simulink model "PIC32MK_MCPWM_MCLV2_PIM_SingleShunt_R2015b_InternalOpAmp"  (R2015b)
settings: Solver=FixedStepDiscrete  StartTime=0.0  StopTime=1  FixedStep=5e-5  RelTol=1e-3
undefined symbols (not defined in the file): A0, A11, A4, AN24, AN25, AN6, AN9, B6, B7, B9, C0, C8, DiscIntNeverNeededParam, G15, MaxPer, ms, Pin, PWM1max, Resol, us, XData
libraries: MCHP_Blockset x14, simulink x9
(part 2 of 3)

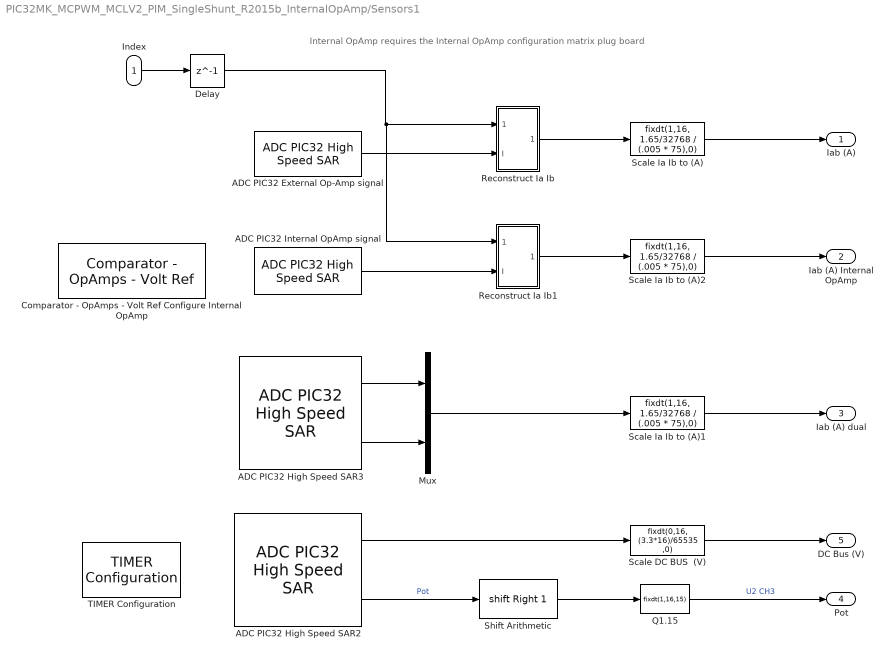
== system PIC32MK_MCPWM_MCLV2_PIM_SingleShunt_R2015b_InternalOpAmp/Sensors1 ==
  note: Internal OpAmp requires the Internal OpAmp configuration matrix plug board
  Index : Inport
  "ADC PIC32 External Op-Amp signal " : MCHP_Blockset/Analog IO/ADC PIC32 High Speed SAR  Priority=-5000  ADC_VrefH=AVdd (default)  ADC_VrefL=AVss (default)  ADC_FRACT=Fractional (left aligned)  DMA_Size=2 trig / 2 elements output (use DMA ping-pong buffer)  ADC_Synchronisation=Triggered by custom source  ADC_Trig=Dynamic Options  ADC_Trig_TXT=PWM1 trigger  ADC_TrigTimeStep=on  ADC_TrigInfo=0  SampleTime=.00005  S_INPUT=[]  S_INPUT_Size=[]  S_OUTPUT=[4]  S_OUTPUT_Size=[2]  S_ListCustomDatatype=S.S_ListCustomDatatype={};  MCHP_USER_INTERRUPTS={AD1D5}{ADC5Data}{ADC Data 5 Ready}{VectorName(ADC_DATA5_VECTOR) Priority(-1) Config_BitSet(ADCGIRQEN1bits.AGIEN5) RegisterReadClear(ADCDATA5)};  MCHP_PORT={Analog Input 25}{AN25}15:2:B7;  MCHP_MASTERLINK=PIC32MK_MCPWM_MCLV2_PIM_SingleShunt_R2015a_InternalOpAmp/Microchip Master  MCHP_CRC=2653067  ADC_Info=Total Time = 450(ns)  ADC0_pin=Dynamic Options  ADC0_pin_TXT=Not used  ADC0_R=< 200 Ohm  ADC0_res=12 bits  ADC0_signed=signed 16 bits  ADC0_FILTER=No Oversampling  ADC0_FILTER_nSamples=8 samples  ADC0_STRGEN=End sampling and start conversion  ADC0_SSAMPEN=on  ADC0_Info=tSmp_min=33.333(ns) x -1 = -33.333(ns) ; tConv=166.67(ns) x 0 = 0(s) ; TOTAL=0(s)  ADC1_pin=Dynamic Options  ADC1_pin_TXT=Not used  ADC1_R=< 200 Ohm  ADC1_res=12 bits  ADC1_signed=signed 16 bits  ADC1_FILTER=No Oversampling  ADC1_FILTER_nSamples=256 samples  ADC1_STRGEN=End sampling and start conversion  ADC1_SSAMPEN=on  ADC1_Info=tSmp_min=33.333(ns) x -1 = -33.333(ns) ; tConv=166.67(ns) x 0 = 0(s) ; TOTAL=0(s)  ADC2_pin=Dynamic Options  ADC2_pin_TXT=Not used  ADC2_R=< 200 Ohm  ADC2_res=12 bits  ADC2_signed=signed 16 bits  ADC2_FILTER=No Oversampling  ADC2_FILTER_nSamples=256 samples  ADC2_STRGEN=End sampling and start conversion  ADC2_SSAMPEN=off  ADC2_Info=tSmp_min=33.333(ns) x -1 = -33.333(ns) ; tConv=166.67(ns) x 0 = 0(s) ; TOTAL=0(s)  ADC3_pin=Dynamic Options  ADC3_pin_TXT=Not used  ADC3_R=< 200 Ohm  ADC3_res=12 bits  ADC3_signed=unsigned 16 bits  ADC3_FILTER=No Oversampling  ADC3_FILTER_nSamples=256 samples  ADC3_STRGEN=End sampling and start conversion  ADC3_SSAMPEN=on  ADC3_Info=tSmp_min=33.333(ns) x -1 = -33.333(ns) ; tConv=166.67(ns) x 0 = 0(s) ; TOTAL=0(s)  ADC4_pin=Dynamic Options  ADC4_pin_TXT=Not used  ADC4_R=< 200 Ohm  ADC4_res=12 bits  ADC4_signed=unsigned 16 bits  ADC4_FILTER=Burst convert of n samples are Averaged  ADC4_FILTER_nSamples=256 samples  ADC4_STRGEN=End sampling and start conversion  ADC4_SSAMPEN=off  ADC4_Info=tSmp_min=33.333(ns) x -1 = -33.333(ns) ; tConv=166.67(ns) x 0 = 0(s) ; TOTAL=0(s)  ADC5_pin=Dynamic Options  ADC5_pin_TXT=AN25 / B7 / Pin[72]  ADC5_R=< 200 Ohm  ADC5_res=12 bits  ADC5_signed=signed 16 bits  ADC5_FILTER=No Oversampling  ADC5_FILTER_nSamples=256 samples  ADC5_STRGEN=End sampling and start conversion  ADC5_SSAMPEN=off  ADC5_Info=tSmp_min=100(ns) x 0 = 0(s) ; tConv=433.33(ns) x 1 = 433.33(ns) ; TOTAL=450(ns)  ADC6_pin=Dynamic Options  ADC6_pin_TXT=Not used  ADC6_R=< 200 Ohm  ADC6_res=12 bits  ADC6_signed=unsigned 16 bits  ADC6_FILTER=Burst convert of n samples are Summed  ADC6_FILTER_nSamples=256 samples  ADC6_STRGEN=End sampling and start conversion  ADC6_SSAMPEN=on  ADC6_Info=tSmp_min=33.333(ns) x -1 = -33.333(ns) ; tConv=166.67(ns) x 0 = 0(s) ; TOTAL=0(s)  ADC7_R=< 200 Ohm  ADC7_res=12 bits  ADC7_AN0=Not used  ADC7_AN1=Not used  ADC7_AN2=Not used  ADC7_AN3=Not used  ADC7_AN4=Not used  ADC7_AN5=Not used  ADC7_AN6=Not used  ADC7_AN7=Not used  ADC7_AN8=Not used  ADC7_AN9=Not used  ADC7_AN10=Not used  ADC7_AN11=Not used  ADC7_AN12=Not used  ADC7_AN13=Not used  ADC7_AN14=Not used  ADC7_AN15=Not used  ADC7_AN16=Not used  ADC7_AN17=Not used  ADC7_AN18=Not used  ADC7_AN19=Not used  ADC7_AN20=Not used  ADC7_AN21=Not used  ADC7_AN22=Not used  ADC7_AN23=Not used  ADC7_AN24=Not used  ADC7_AN25=Not used  ADC7_AN26=Not used  ADC7_AN27=Not used  ADC7_AN28=Not used  ADC7_AN29=Not used  ADC7_AN30=Not used  ADC7_AN31=Not used  ADC7_AN32=Not used  ADC7_AN33=Not used  ADC7_AN34=Not used  ADC7_AN35=Not used  ADC7_AN36=Not used  ADC7_AN37=Not used  ADC7_AN38=Not used  ADC7_AN39=Not used  ADC7_AN40=Not used  ADC7_AN41=Not used  ADC7_AN42=Not used  ADC7_AN43=Not used  ADC7_AN44=Not used  ADC7_AN45=Not used  ADC7_AN46=Not used  ADC7_AN47=Not used  ADC7_AN48=Not used  ADC7_AN49=Not used  ADC7_AN50=Not used  ADC7_AN51=Not used  ADC7_AN52=Not used  ADC7_AN53=Not used  ADC7_AN54=Not used  ADC7_AN55=Not used  ADC7_AN56=Not used  ADC7_AN57=Not used  ADC7_AN58=Not used  ADC7_AN59=Not used  ADC7_AN60=Not used  ADC7_AN61=Not used  ADC7_AN62=Not used  ADC7_AN63=Not used  CTMU_Temp=Not used  Vbat=Not used  IVref=Not used  IVTemp=Not used
  ADC PIC32 High Speed SAR2 : MCHP_Blockset/Analog IO/ADC PIC32 High Speed SAR  Priority=-5000  ADC_VrefH=AVdd (default)  ADC_VrefL=AVss (default)  ADC_FRACT=Fractional (left aligned)  DMA_Size=Single trigger - (no DMA)  ADC_Synchronisation=Triggered by custom source  ADC_Trig=Dynamic Options  ADC_Trig_TXT=TMR5 Match  ADC_TrigTimeStep=off  ADC_TrigInfo=0  SampleTime=.001  S_INPUT=[]  S_INPUT_Size=[]  S_OUTPUT="[5  5]"  S_OUTPUT_Size="[1  1]"  S_ListCustomDatatype=S.S_ListCustomDatatype={};  MCHP_USER_INTERRUPTS={AD1D9}{ADC9Data}{ADC Data 9 Ready}{VectorName(ADC_DATA9_VECTOR) Priority(-1) Config_BitSet(ADCGIRQEN1bits.AGIEN9) RegisterReadClear(ADCDATA9)};{AD1D14}{ADC14Data}{ADC Data 14 Ready}{VectorName(ADC_DATA14_VECTOR) Priority(-1) Config_BitSet(ADCGIRQEN1bits.AGIEN14) RegisterReadClear(ADCDATA14)};  MCHP_PORT={Analog Input 10}{AN10}15:2:A12;{Analog Input 15}{AN15}15:2:E15;  MCHP_MASTERLINK=PIC32MK_MCPWM_MCLV2_PIM_SingleShunt_R2015a_InternalOpAmp/Microchip Master  MCHP_CRC=2878404  ADC_Info=Total Time = 149.917(us)  ADC0_pin=Dynamic Options  ADC0_pin_TXT=Not used  ADC0_R=< 200 Ohm  ADC0_res=12 bits  ADC0_signed=signed 16 bits  ADC0_FILTER=No Oversampling  ADC0_FILTER_nSamples=256 samples  ADC0_STRGEN=End sampling and start conversion  ADC0_SSAMPEN=on  ADC0_Info=tSmp_min=33.333(ns) x -1 = -33.333(ns) ; tConv=166.67(ns) x 0 = 0(s) ; TOTAL=0(s)  ADC1_pin=Dynamic Options  ADC1_pin_TXT=Not used  ADC1_R=< 200 Ohm  ADC1_res=12 bits  ADC1_signed=signed 16 bits  ADC1_FILTER=No Oversampling  ADC1_FILTER_nSamples=256 samples  ADC1_STRGEN=End sampling and start conversion  ADC1_SSAMPEN=on  ADC1_Info=tSmp_min=33.333(ns) x -1 = -33.333(ns) ; tConv=166.67(ns) x 0 = 0(s) ; TOTAL=0(s)  ADC2_pin=Dynamic Options  ADC2_pin_TXT=Not used  ADC2_R=< 200 Ohm  ADC2_res=12 bits  ADC2_signed=signed 16 bits  ADC2_FILTER=Burst convert of n samples are Summed  ADC2_FILTER_nSamples=256 samples  ADC2_STRGEN=End sampling and start conversion  ADC2_SSAMPEN=off  ADC2_Info=tSmp_min=33.333(ns) x -1 = -33.333(ns) ; tConv=166.67(ns) x 0 = 0(s) ; TOTAL=0(s)  ADC3_pin=Dynamic Options  ADC3_pin_TXT=Not used  ADC3_R=< 200 Ohm  ADC3_res=12 bits  ADC3_signed=unsigned 16 bits  ADC3_FILTER=No Oversampling  ADC3_FILTER_nSamples=256 samples  ADC3_STRGEN=End sampling and start conversion  ADC3_SSAMPEN=on  ADC3_Info=tSmp_min=33.333(ns) x -1 = -33.333(ns) ; tConv=166.67(ns) x 0 = 0(s) ; TOTAL=0(s)  ADC4_pin=Dynamic Options  ADC4_pin_TXT=Not used  ADC4_R=< 200 Ohm  ADC4_res=12 bits  ADC4_signed=unsigned 16 bits  ADC4_FILTER=Burst convert of n samples are Averaged  ADC4_FILTER_nSamples=256 samples  ADC4_STRGEN=End sampling and start conversion  ADC4_SSAMPEN=off  ADC4_Info=tSmp_min=33.333(ns) x -1 = -33.333(ns) ; tConv=166.67(ns) x 0 = 0(s) ; TOTAL=0(s)  ADC5_pin=Dynamic Options  ADC5_pin_TXT=Not used  ADC5_R=< 200 Ohm  ADC5_res=12 bits  ADC5_signed=unsigned 16 bits  ADC5_FILTER=No Oversampling  ADC5_FILTER_nSamples=256 samples  ADC5_STRGEN=End sampling and start conversion  ADC5_SSAMPEN=off  ADC5_Info=tSmp_min=33.333(ns) x -1 = -33.333(ns) ; tConv=166.67(ns) x 0 = 0(s) ; TOTAL=0(s)  ADC6_pin=Dynamic Options  ADC6_pin_TXT=Not used  ADC6_R=< 200 Ohm  ADC6_res=12 bits  ADC6_signed=unsigned 16 bits  ADC6_FILTER=Burst convert of n samples are Summed  ADC6_FILTER_nSamples=256 samples  ADC6_STRGEN=End sampling and start conversion  ADC6_SSAMPEN=on  ADC6_Info=tSmp_min=33.333(ns) x -1 = -33.333(ns) ; tConv=166.67(ns) x 0 = 0(s) ; TOTAL=0(s)  ADC7_R=< 200 Ohm  ADC7_res=12 bits  ADC7_AN0=Not used  ADC7_AN1=Not used  ADC7_AN2=Not used  ADC7_AN3=Not used  ADC7_AN4=Not used  ADC7_AN5=Not used  ADC7_AN6=Not used  ADC7_AN7=Not used  ADC7_AN8=Not used  ADC7_AN9=Not used  ADC7_AN10=unsigned int16  ADC7_AN11=Not used  ADC7_AN12=Not used  ADC7_AN13=Not used  ADC7_AN14=Not used  ADC7_AN15=256 samples averaged - unsigned int16  ADC7_AN16=Not used  ADC7_AN17=Not used  ADC7_AN18=Not used  ADC7_AN19=Not used  ADC7_AN20=Not used  ADC7_AN21=Not used  ADC7_AN22=Not used  ADC7_AN23=Not used  ADC7_AN24=Not used  ADC7_AN25=Not used  ADC7_AN26=Not used  ADC7_AN27=Not used  ADC7_AN28=Not used  ADC7_AN29=Not used  ADC7_AN30=Not used  ADC7_AN31=Not used  ADC7_AN32=Not used  ADC7_AN33=Not used  ADC7_AN34=Not used  ADC7_AN35=Not used  ADC7_AN36=Not used  ADC7_AN37=Not used  ADC7_AN38=Not used  ADC7_AN39=Not used  ADC7_AN40=Not used  ADC7_AN41=Not used  ADC7_AN42=Not used  ADC7_AN43=Not used  ADC7_AN44=Not used  ADC7_AN45=Not used  ADC7_AN46=Not used  ADC7_AN47=Not used  ADC7_AN48=Not used  ADC7_AN49=Not used  ADC7_AN50=Not used  ADC7_AN51=Not used  ADC7_AN52=Not used  ADC7_AN53=Not used  ADC7_AN54=Not used  ADC7_AN55=Not used  ADC7_AN56=Not used  ADC7_AN57=Not used  ADC7_AN58=Not used  ADC7_AN59=Not used  ADC7_AN60=Not used  ADC7_AN61=Not used  ADC7_AN62=Not used  ADC7_AN63=Not used  CTMU_Temp=Not used  Vbat=Not used  IVref=Not used  IVTemp=Not used
  ADC PIC32 High Speed SAR3 : MCHP_Blockset/Analog IO/ADC PIC32 High Speed SAR  Priority=-5000  ADC_VrefH=AVdd (default)  ADC_VrefL=AVss (default)  ADC_FRACT=Fractional (left aligned)  DMA_Size=Single trigger - (no DMA)  ADC_Synchronisation=Triggered by custom source  ADC_Trig=Dynamic Options  ADC_Trig_TXT=PWM2 trigger  ADC_TrigTimeStep=off  ADC_TrigInfo=0  SampleTime=.00005  S_INPUT=[]  S_INPUT_Size=[]  S_OUTPUT="[4  4]"  S_OUTPUT_Size="[1  1]"  S_ListCustomDatatype=S.S_ListCustomDatatype={};  MCHP_USER_INTERRUPTS={AD1D0}{ADC0Data}{ADC Data 0 Ready}{VectorName(ADC_DATA0_VECTOR) Priority(-1) Config_BitSet(ADCGIRQEN1bits.AGIEN0) RegisterReadClear(ADCDATA0)};{AD1D4}{ADC4Data}{ADC Data 4 Ready}{VectorName(ADC_DATA4_VECTOR) Priority(-1) Config_BitSet(ADCGIRQEN1bits.AGIEN4) RegisterReadClear(ADCDATA4)};  MCHP_PORT={Analog Input 24}{AN24}15:2:A4;{Analog Input 9}{AN9}15:2:A11;  MCHP_MASTERLINK=PIC32MK_MCPWM_MCLV2_PIM_SingleShunt_R2015a_InternalOpAmp/Microchip Master  MCHP_CRC=2708506  ADC_Info=Total Time = 450(ns)  ADC0_pin=Dynamic Options  ADC0_pin_TXT=AN24 / A4 / Pin[51]  ADC0_R=< 200 Ohm  ADC0_res=12 bits  ADC0_signed=signed 16 bits  ADC0_FILTER=No Oversampling  ADC0_FILTER_nSamples=8 samples  ADC0_STRGEN=End sampling and start conversion  ADC0_SSAMPEN=on  ADC0_Info=tSmp_min=100(ns) x 0 = 0(s) ; tConv=433.33(ns) x 1 = 433.33(ns) ; TOTAL=450(ns)  ADC1_pin=Dynamic Options  ADC1_pin_TXT=Not used  ADC1_R=< 200 Ohm  ADC1_res=12 bits  ADC1_signed=signed 16 bits  ADC1_FILTER=No Oversampling  ADC1_FILTER_nSamples=256 samples  ADC1_STRGEN=End sampling and start conversion  ADC1_SSAMPEN=on  ADC1_Info=tSmp_min=33.333(ns) x -1 = -33.333(ns) ; tConv=166.67(ns) x 0 = 0(s) ; TOTAL=0(s)  ADC2_pin=Dynamic Options  ADC2_pin_TXT=Not used  ADC2_R=< 200 Ohm  ADC2_res=12 bits  ADC2_signed=signed 16 bits  ADC2_FILTER=No Oversampling  ADC2_FILTER_nSamples=256 samples  ADC2_STRGEN=End sampling and start conversion  ADC2_SSAMPEN=on  ADC2_Info=tSmp_min=33.333(ns) x -1 = -33.333(ns) ; tConv=166.67(ns) x 0 = 0(s) ; TOTAL=0(s)  ADC3_pin=Dynamic Options  ADC3_pin_TXT=Not used  ADC3_R=< 200 Ohm  ADC3_res=12 bits  ADC3_signed=unsigned 16 bits  ADC3_FILTER=No Oversampling  ADC3_FILTER_nSamples=256 samples  ADC3_STRGEN=End sampling and start conversion  ADC3_SSAMPEN=on  ADC3_Info=tSmp_min=33.333(ns) x -1 = -33.333(ns) ; tConv=166.67(ns) x 0 = 0(s) ; TOTAL=0(s)  ADC4_pin=Dynamic Options  ADC4_pin_TXT=AN9 / A11 / Pin[21]  ADC4_R=< 200 Ohm  ADC4_res=12 bits  ADC4_signed=signed 16 bits  ADC4_FILTER=No Oversampling  ADC4_FILTER_nSamples=256 samples  ADC4_STRGEN=End sampling and start conversion  ADC4_SSAMPEN=on  ADC4_Info=tSmp_min=100(ns) x 0 = 0(s) ; tConv=433.33(ns) x 1 = 433.33(ns) ; TOTAL=450(ns)  ADC5_pin=Dynamic Options  ADC5_pin_TXT=Not used  ADC5_R=< 200 Ohm  ADC5_res=12 bits  ADC5_signed=unsigned 16 bits  ADC5_FILTER=No Oversampling  ADC5_FILTER_nSamples=256 samples  ADC5_STRGEN=End sampling and start conversion  ADC5_SSAMPEN=off  ADC5_Info=tSmp_min=33.333(ns) x -1 = -33.333(ns) ; tConv=166.67(ns) x 0 = 0(s) ; TOTAL=0(s)  ADC6_pin=Dynamic Options  ADC6_pin_TXT=Not used  ADC6_R=< 200 Ohm  ADC6_res=12 bits  ADC6_signed=unsigned 16 bits  ADC6_FILTER=Burst convert of n samples are Summed  ADC6_FILTER_nSamples=256 samples  ADC6_STRGEN=End sampling and start conversion  ADC6_SSAMPEN=on  ADC6_Info=tSmp_min=33.333(ns) x -1 = -33.333(ns) ; tConv=166.67(ns) x 0 = 0(s) ; TOTAL=0(s)  ADC7_R=< 200 Ohm  ADC7_res=12 bits  ADC7_AN0=Not used  ADC7_AN1=Not used  ADC7_AN2=Not used  ADC7_AN3=Not used  ADC7_AN4=Not used  ADC7_AN5=Not used  ADC7_AN6=Not used  ADC7_AN7=Not used  ADC7_AN8=Not used  ADC7_AN9=Not used  ADC7_AN10=Not used  ADC7_AN11=Not used  ADC7_AN12=Not used  ADC7_AN13=Not used  ADC7_AN14=Not used  ADC7_AN15=Not used  ADC7_AN16=Not used  ADC7_AN17=Not used  ADC7_AN18=Not used  ADC7_AN19=Not used  ADC7_AN20=Not used  ADC7_AN21=Not used  ADC7_AN22=Not used  ADC7_AN23=Not used  ADC7_AN24=Not used  ADC7_AN25=Not used  ADC7_AN26=Not used  ADC7_AN27=Not used  ADC7_AN28=Not used  ADC7_AN29=Not used  ADC7_AN30=Not used  ADC7_AN31=Not used  ADC7_AN32=Not used  ADC7_AN33=Not used  ADC7_AN34=Not used  ADC7_AN35=Not used  ADC7_AN36=Not used  ADC7_AN37=Not used  ADC7_AN38=Not used  ADC7_AN39=Not used  ADC7_AN40=Not used  ADC7_AN41=Not used  ADC7_AN42=Not used  ADC7_AN43=Not used  ADC7_AN44=Not used  ADC7_AN45=Not used  ADC7_AN46=Not used  ADC7_AN47=Not used  ADC7_AN48=Not used  ADC7_AN49=Not used  ADC7_AN50=Not used  ADC7_AN51=Not used  ADC7_AN52=Not used  ADC7_AN53=Not used  ADC7_AN54=Not used  ADC7_AN55=Not used  ADC7_AN56=Not used  ADC7_AN57=Not used  ADC7_AN58=Not used  ADC7_AN59=Not used  ADC7_AN60=Not used  ADC7_AN61=Not used  ADC7_AN62=Not used  ADC7_AN63=Not used  CTMU_Temp=Not used  Vbat=Not used  IVref=Not used  IVTemp=Not used
  ADC PIC32 Internal OpAmp signal : MCHP_Blockset/Analog IO/ADC PIC32 High Speed SAR  Priority=-5000  ADC_VrefH=AVdd (default)  ADC_VrefL=AVss (default)  ADC_FRACT=Fractional (left aligned)  DMA_Size=2 trig / 2 elements output (use DMA ping-pong buffer)  ADC_Synchronisation=Triggered by custom source  ADC_Trig=Dynamic Options  ADC_Trig_TXT=PWM1 trigger  ADC_TrigTimeStep=on  ADC_TrigInfo=0  SampleTime=.00005  S_INPUT=[]  S_INPUT_Size=[]  S_OUTPUT=[4]  S_OUTPUT_Size=[2]  S_ListCustomDatatype=S.S_ListCustomDatatype={};  MCHP_USER_INTERRUPTS={AD1D2}{ADC2Data}{ADC Data 2 Ready}{VectorName(ADC_DATA2_VECTOR) Priority(-1) Config_BitSet(ADCGIRQEN1bits.AGIEN2) RegisterReadClear(ADCDATA2)};  MCHP_PORT={Analog Input 6}{AN6}15:2:C0;  MCHP_MASTERLINK=PIC32MK_MCPWM_MCLV2_PIM_SingleShunt_R2015a_InternalOpAmp/Microchip Master  MCHP_CRC=2657833  ADC_Info=Total Time = 450(ns)  ADC0_pin=Dynamic Options  ADC0_pin_TXT=Not used  ADC0_R=< 200 Ohm  ADC0_res=12 bits  ADC0_signed=signed 16 bits  ADC0_FILTER=No Oversampling  ADC0_FILTER_nSamples=8 samples  ADC0_STRGEN=End sampling and start conversion  ADC0_SSAMPEN=on  ADC0_Info=tSmp_min=33.333(ns) x -1 = -33.333(ns) ; tConv=166.67(ns) x 0 = 0(s) ; TOTAL=0(s)  ADC1_pin=Dynamic Options  ADC1_pin_TXT=Not used  ADC1_R=< 200 Ohm  ADC1_res=12 bits  ADC1_signed=signed 16 bits  ADC1_FILTER=No Oversampling  ADC1_FILTER_nSamples=256 samples  ADC1_STRGEN=End sampling and start conversion  ADC1_SSAMPEN=on  ADC1_Info=tSmp_min=33.333(ns) x -1 = -33.333(ns) ; tConv=166.67(ns) x 0 = 0(s) ; TOTAL=0(s)  ADC2_pin=Dynamic Options  ADC2_pin_TXT=AN6 / C0 / Pin[32]  ADC2_R=< 200 Ohm  ADC2_res=12 bits  ADC2_signed=signed 16 bits  ADC2_FILTER=No Oversampling  ADC2_FILTER_nSamples=256 samples  ADC2_STRGEN=End sampling and start conversion  ADC2_SSAMPEN=off  ADC2_Info=tSmp_min=100(ns) x 0 = 0(s) ; tConv=433.33(ns) x 1 = 433.33(ns) ; TOTAL=450(ns)  ADC3_pin=Dynamic Options  ADC3_pin_TXT=Not used  ADC3_R=< 200 Ohm  ADC3_res=12 bits  ADC3_signed=unsigned 16 bits  ADC3_FILTER=No Oversampling  ADC3_FILTER_nSamples=256 samples  ADC3_STRGEN=End sampling and start conversion  ADC3_SSAMPEN=on  ADC3_Info=tSmp_min=33.333(ns) x -1 = -33.333(ns) ; tConv=166.67(ns) x 0 = 0(s) ; TOTAL=0(s)  ADC4_pin=Dynamic Options  ADC4_pin_TXT=Not used  ADC4_R=< 200 Ohm  ADC4_res=12 bits  ADC4_signed=unsigned 16 bits  ADC4_FILTER=Burst convert of n samples are Averaged  ADC4_FILTER_nSamples=256 samples  ADC4_STRGEN=End sampling and start conversion  ADC4_SSAMPEN=off  ADC4_Info=tSmp_min=33.333(ns) x -1 = -33.333(ns) ; tConv=166.67(ns) x 0 = 0(s) ; TOTAL=0(s)  ADC5_pin=Dynamic Options  ADC5_pin_TXT=Not used  ADC5_R=< 200 Ohm  ADC5_res=12 bits  ADC5_signed=signed 16 bits  ADC5_FILTER=No Oversampling  ADC5_FILTER_nSamples=256 samples  ADC5_STRGEN=End sampling and start conversion  ADC5_SSAMPEN=off  ADC5_Info=tSmp_min=33.333(ns) x -1 = -33.333(ns) ; tConv=166.67(ns) x 0 = 0(s) ; TOTAL=0(s)  ADC6_pin=Dynamic Options  ADC6_pin_TXT=Not used  ADC6_R=< 200 Ohm  ADC6_res=12 bits  ADC6_signed=unsigned 16 bits  ADC6_FILTER=Burst convert of n samples are Summed  ADC6_FILTER_nSamples=256 samples  ADC6_STRGEN=End sampling and start conversion  ADC6_SSAMPEN=on  ADC6_Info=tSmp_min=33.333(ns) x -1 = -33.333(ns) ; tConv=166.67(ns) x 0 = 0(s) ; TOTAL=0(s)  ADC7_R=< 200 Ohm  ADC7_res=12 bits  ADC7_AN0=Not used  ADC7_AN1=Not used  ADC7_AN2=Not used  ADC7_AN3=Not used  ADC7_AN4=Not used  ADC7_AN5=Not used  ADC7_AN6=Not used  ADC7_AN7=Not used  ADC7_AN8=Not used  ADC7_AN9=Not used  ADC7_AN10=Not used  ADC7_AN11=Not used  ADC7_AN12=Not used  ADC7_AN13=Not used  ADC7_AN14=Not used  ADC7_AN15=Not used  ADC7_AN16=Not used  ADC7_AN17=Not used  ADC7_AN18=Not used  ADC7_AN19=Not used  ADC7_AN20=Not used  ADC7_AN21=Not used  ADC7_AN22=Not used  ADC7_AN23=Not used  ADC7_AN24=Not used  ADC7_AN25=Not used  ADC7_AN26=Not used  ADC7_AN27=Not used  ADC7_AN28=Not used  ADC7_AN29=Not used  ADC7_AN30=Not used  ADC7_AN31=Not used  ADC7_AN32=Not used  ADC7_AN33=Not used  ADC7_AN34=Not used  ADC7_AN35=Not used  ADC7_AN36=Not used  ADC7_AN37=Not used  ADC7_AN38=Not used  ADC7_AN39=Not used  ADC7_AN40=Not used  ADC7_AN41=Not used  ADC7_AN42=Not used  ADC7_AN43=Not used  ADC7_AN44=Not used  ADC7_AN45=Not used  ADC7_AN46=Not used  ADC7_AN47=Not used  ADC7_AN48=Not used  ADC7_AN49=Not used  ADC7_AN50=Not used  ADC7_AN51=Not used  ADC7_AN52=Not used  ADC7_AN53=Not used  ADC7_AN54=Not used  ADC7_AN55=Not used  ADC7_AN56=Not used  ADC7_AN57=Not used  ADC7_AN58=Not used  ADC7_AN59=Not used  ADC7_AN60=Not used  ADC7_AN61=Not used  ADC7_AN62=Not used  ADC7_AN63=Not used  CTMU_Temp=Not used  Vbat=Not used  IVref=Not used  IVTemp=Not used
  Comparator - OpAmps - Volt Ref Configure Internal OpAmp : MCHP_Blockset/Analog IO/Comparator - OpAmps - Volt Ref  MCHP_params=s.CVR1OE=0;s.CVR2OE=1;s.VREFSEL=0;s.RLaddle=reshape([1 1889],1,2);s.AVdd=reshape({ '3.3','3.3'},1,2);s.AVss=reshape({ '0','0'},1,2);s.CVRSS=reshape([0 0],1,2);s.CON_OPMODE_CPOL=reshape([0 0 3 0 0],1,5);s.OutputPort_COE_RP=reshape({ 'None','None','C0 / Pin[32] / OA3OUT / AN6 / OA3OUT','None','None'},1,5);s.InputP_CREF=reshape([0 0 0 0 0],1,5);s.InputN_CCH=reshape([0 0 0 0 0],1,5);s.Trigger_EventInterrupt_EVPOL=reshape([0 0 0 0 0],1,5);s.BlockOutputEvent=reshape([0 0 0 0 0],1,5);s.BlockOutputState=reshape([0 0 0 0 0],1,5);s.IntPriority=5;s.FilterFreq=reshape([1e+10 1e+10 1e+10 1e+10 1e+10],1,5);s.Blanking=reshape([1 1 1 1 1],1,5);s.BlankingSignal=reshape({ ' - ',' - ',' - ',' - ',' - ',' - ',' - ',' - ',' - ',' - ',' - ',' - ',' - ',' - ',' - '},3,5);s.BlankingTruthTable=reshape([-1 -1 -1 -1 -1 -1 -1 -1 -1 -1 -1 -1 -1 -1 -1 -1 -1 -1 -1 -1 -1 -1 -1 -1 -1 -1 -1 -1 -1 -1 -1 -1 -1 -1 -1 -1 -1 -1 -1 -1 -1 -1 -1 -1 -1 -1 -1 -1 -1 -1 -1 -1 -1 -1 -1 -1 -1 -1 -1 -1 -1 -1 -1 -1 -1 -1 -1 -1 -1 -1 -1 -1 -1 -1 -1 -1 -1 -1 -1 -1 -1 -1 -1 -1 -1 -1 -1 -1 -1 -1 -1 -1 -1 -1 -1 -1 -1 -1 -1 -1 -1 -1 -1 -1 -1 -1 -1 -1 -1 -1 -1 -1 -1 -1 -1 -1 -1 -1 -1 -1 -1 -1 -1 -1 -1 -1 -1 -1 -1 -1 -1 -1 -1 -1 -1 -1 -1 -1 -1 -1 -1 -1 -1 -1 -1 -1 -1 -1 -1 -1 -1 -1 -1 -1 -1 -1 -1 -1 -1 -1 -1 -1 -1 -1 -1 -1 -1 -1 -1 -1 -1 -1 -1 -1 -1 -1 -1 -1 -1 -1 -1 -1 -1 -1 -1 -1 -1 -1 -1 -1 -1 -1 -1 -1 -1 -1 -1 -1 -1 -1 -1 -1 -1 -1 -1 -1 -1 -1 -1 -1 -1 -1 -1 -1 -1 -1 -1 -1 -1 -1 -1 -1 -1 -1 -1 -1 -1 -1 -1 -1 -1 -1 -1 -1 -1 -1 -1 -1 -1 -1],16 ,3 ,5);  S_INPUT="[5  5]"  S_OUTPUT=[5]  S_INPUT_Size="[2  2]"  S_OUTPUT_Size=[4]  SampleTime=-1  MCHP_MASTERLINK=PIC32MK_MCPWM_MCLV2_PIM_SingleShunt_R2015a_InternalOpAmp/Microchip Master  MCHP_PORT={Comparator Output Reference 2}{CVref2O}14:2:C10;{Op-Amp Output 3}{OA3(out)}14:2:C0;{Op-Amp3 V+}{OA3 V+}14:2:C2;{Op-Amp3 V-}{OA3 V-}14:2:C1;  ORDERING=0
  Delay : Delay  DelayLength=1  InitialCondition=0
  Mux : Mux  Inputs=2
  Q1.15 : DataTypeConversion  OutDataTypeStr=fixdt(1,16,15)  ConvertRealWorld=Stored Integer (SI)
  Reconstruct Ia Ib : Subsystem  AncestorBlock=|
      | Lib_MCHP_BLKDEMO_Motor/MOTOR/SINGLE SHUNT
      | Center Aligned/MOTOR - Board
      | Sensor/Reconstruct
      | Ia Ib
  Reconstruct Ia Ib1 : Subsystem  AncestorBlock=|
      | Lib_MCHP_BLKDEMO_Motor/MOTOR/SINGLE SHUNT
      | Center Aligned/MOTOR - Board
      | Sensor/Reconstruct
      | Ia Ib
  Scale DC BUS  (V) : DataTypeConversion  OutDataTypeStr=fixdt(0,16, (3.3*16)/65535 ,0)  ConvertRealWorld=Stored Integer (SI)
  Scale Ia Ib to (A) : DataTypeConversion  OutDataTypeStr=fixdt(1,16, 1.65/32768 / (.005 * 75),0)  ConvertRealWorld=Stored Integer (SI)
  Scale Ia Ib to (A)1 : DataTypeConversion  OutDataTypeStr=fixdt(1,16, 1.65/32768 / (.005 * 75),0)  ConvertRealWorld=Stored Integer (SI)
  Scale Ia Ib to (A)2 : DataTypeConversion  OutDataTypeStr=fixdt(1,16, 1.65/32768 / (.005 * 75),0)  ConvertRealWorld=Stored Integer (SI)
  Shift Arithmetic : ArithShift  BitShiftNumber=1  BitShiftDirection=Right
  TIMER Configuration : MCHP_Blockset/Timers/TIMER Configuration  TIMER_Name=TimerB  TIMER_CustomName=pouet_p  TIMER_Ressource=Dynamic Options  TIMER_Ressource_TXT=Timer 5  TIMER_Ressource_Custom=[1]  DoNotSetupChk=off  TIMER_PeriodChk=off  TIMER_Period=1e-3  TIMER_Resolution=Dynamic Options  TIMER_Resolution_TXT="Resol: 0.008333(us)  -  MaxPer: 0.546(ms)"  TIMER_Interrupt=off  TIMER_Use=Read only  TIMER_ShareChk=on  MCHP_TIMER_REQUEST={TimerB}{TmrCfg}20:2:3:0:[5]:120000;  MCHP_TIMER_RESULT=[5 59998.999999999971 ]  MCHP_USER_INTERRUPTS={T5}{TimerB}{TimerB}{VectorName(TIMER_5_VECTOR) Priority(-1) };  MCHP_MASTERLINK=PIC32MK_MCPWM_MCLV2_PIM_SingleShunt_R2015a_InternalOpAmp/Microchip Master  Info="Timer 5:  Resol: 16.66666667(ns)  -  Per: 1(ms)  -  Max value: 1.09225(ms)"
  Iab (A) : Outport
  Iab (A) Internal OpAmp : Outport  Port=2
  Iab (A) dual : Outport  Port=3
  Pot : Outport  Port=4
  DC Bus (V) : Outport  Port=5
  wires:
  Scale DC BUS  (V)/1 -> DC Bus (V)/1
  Scale Ia Ib to (A)/1 -> Iab (A)/1
  Q1.15/1 -> Pot/1  "U2 CH3"
  ADC PIC32 High Speed SAR2/2 -> Shift Arithmetic/1  "Pot"
  "ADC PIC32 External Op-Amp signal "/1 -> Reconstruct Ia Ib/2(I)
  Delay/1 -> Reconstruct Ia Ib1/1(Index), Reconstruct Ia Ib/1(Index)
  Index/1 -> Delay/1
  Reconstruct Ia Ib/1(Ia Ib) -> Scale Ia Ib to (A)/1
  Scale Ia Ib to (A)1/1 -> Iab (A) dual/1
  ADC PIC32 High Speed SAR3/1 -> Mux/1
  ADC PIC32 High Speed SAR3/2 -> Mux/2
  Mux/1 -> Scale Ia Ib to (A)1/1
  ADC PIC32 High Speed SAR2/1 -> Scale DC BUS  (V)/1
  Shift Arithmetic/1 -> Q1.15/1
  ADC PIC32 Internal OpAmp signal/1 -> Reconstruct Ia Ib1/2(I)
  Reconstruct Ia Ib1/1(Ia Ib) -> Scale Ia Ib to (A)2/1
  Scale Ia Ib to (A)2/1 -> Iab (A) Internal OpAmp/1

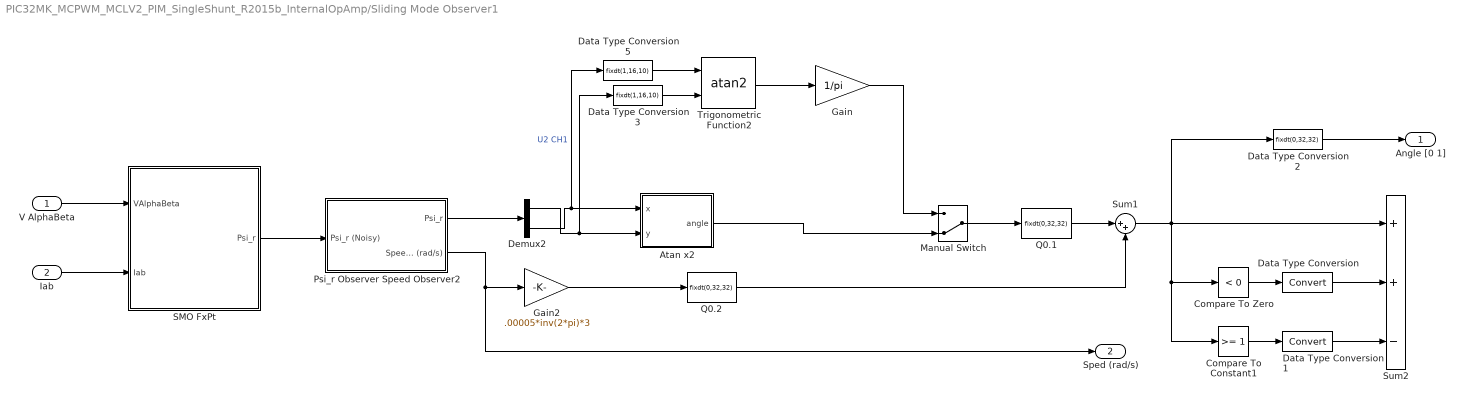
== system PIC32MK_MCPWM_MCLV2_PIM_SingleShunt_R2015b_InternalOpAmp/Sliding Mode Observer1 ==
  V AlphaBeta : Inport
  Iab : Inport  Port=2
  Atan x2 : Subsystem  AncestorBlock=Lib_MCHP_BLKDEMO_Motor/Atan x2
  Compare To Constant1 : simulink/Logic and Bit Operations/Compare To Constant  relop=>=  const=1  OutDataTypeStr=boolean
  Compare To Zero : simulink/Logic and Bit Operations/Compare To Zero  relop=<  OutDataTypeStr=boolean
  Data Type Conversion : DataTypeConversion  RndMeth=Zero
  Data Type Conversion1 : DataTypeConversion  RndMeth=Zero
  Data Type Conversion2 : DataTypeConversion  OutDataTypeStr=fixdt(0,32,32)  RndMeth=Zero
  Data Type Conversion3 : DataTypeConversion  OutDataTypeStr=fixdt(1,16,10)  RndMeth=Zero
  Data Type Conversion5 : DataTypeConversion  OutDataTypeStr=fixdt(1,16,10)  RndMeth=Zero
  Demux2 : Demux  Outputs=2
  Gain : Gain  Gain=1/pi  OutDataTypeStr=fixdt(1,32,31)  RndMeth=Zero
  Gain2 : Gain  Gain=.00005*inv(2*pi)*3  OutDataTypeStr=fixdt(1,32,31)  RndMeth=Zero
  Manual Switch : ManualSwitch  CurrentSetting=0
  Psi_r Observer Speed Observer2 : Subsystem
  Q0.1 : DataTypeConversion  OutDataTypeStr=fixdt(0,32,32)  ConvertRealWorld=Stored Integer (SI)  RndMeth=Simplest
  Q0.2 : DataTypeConversion  OutDataTypeStr=fixdt(0,32,32)  ConvertRealWorld=Stored Integer (SI)  RndMeth=Simplest
  SMO FxPt : Subsystem
  Sum1 : Sum  Inputs=|++  OutDataTypeStr=Inherit: Same as accumulator  RndMeth=Zero
  Sum2 : Sum  Inputs=++-  OutDataTypeStr=Inherit: Same as accumulator  RndMeth=Zero
  Trigonometric Function2 : Trigonometry  Operator=atan2  ApproximationMethod=CORDIC  NumberOfIterations=10  OutputSignalType=real
  Angle [0 1] : Outport
  Sped (rad/s) : Outport  Port=2
  wires:
  Data Type Conversion2/1 -> Angle [0 1]/1
  Trigonometric Function2/1 -> Gain/1
  Data Type Conversion1/1 -> Sum2/3
  Data Type Conversion/1 -> Sum2/2
  Compare To Constant1/1 -> Data Type Conversion1/1
  Compare To Zero/1 -> Data Type Conversion/1
  Gain/1 -> Manual Switch/1
  Atan x2/1(angle) -> Manual Switch/2
  Demux2/2 -> Data Type Conversion5/1, Atan x2/1(x)  "U2 CH1"
  Manual Switch/1 -> Q0.1/1
  Sum1/1 -> Compare To Zero/1, Compare To Constant1/1, Data Type Conversion2/1, Sum2/1
  Iab/1 -> SMO FxPt/2(Iab)
  Psi_r Observer Speed Observer2/2(Speed we (rad/s)) -> Gain2/1, Sped (rad/s)/1
  SMO FxPt/1(Psi_r) -> Psi_r Observer Speed Observer2/1(Psi_r (Noisy))
  V AlphaBeta/1 -> SMO FxPt/1(VAlphaBeta)
  Psi_r Observer Speed Observer2/1(Psi_r) -> Demux2/1
  Demux2/1 -> Atan x2/2(y), Data Type Conversion3/1
  Gain2/1 -> Q0.2/1
  Q0.1/1 -> Sum1/1
  Data Type Conversion5/1 -> Trigonometric Function2/1
  Data Type Conversion3/1 -> Trigonometric Function2/2
  Q0.2/1 -> Sum1/2

== system PIC32MK_MCPWM_MCLV2_PIM_SingleShunt_R2015b_InternalOpAmp/Subsystem1 ==
  OL : Inport
  CL : Inport  Port=2
  Rate Transition10 : RateTransition
  Switch Startup ramp Angle then Estimated Angle or QEI : Switch  Criteria=u2 ~= 0  Threshold=250
  OL/CL : Outport
  wires:
  [CL] -> Rate Transition10/1
  Rate Transition10/1 -> Switch Startup ramp Angle then Estimated Angle or QEI/2
  Switch Startup ramp Angle then Estimated Angle or QEI/1 -> OL/CL/1
  OL/1 -> Switch Startup ramp Angle then Estimated Angle or QEI/3
  CL/1 -> Switch Startup ramp Angle then Estimated Angle or QEI/1

== system PIC32MK_MCPWM_MCLV2_PIM_SingleShunt_R2015b_InternalOpAmp/Subsystem2 ==
  CL : Inport
  OL : Inport  Port=2
  Rate Transition10 : RateTransition
  Switch Startup ramp Angle then Estimated Angle or QEI : Switch  Criteria=u2 ~= 0  Threshold=250
  OL/CL : Outport
  wires:
  CL/1 -> Switch Startup ramp Angle then Estimated Angle or QEI/1
  OL/1 -> Switch Startup ramp Angle then Estimated Angle or QEI/3
  Rate Transition10/1 -> Switch Startup ramp Angle then Estimated Angle or QEI/2
  [CL] -> Rate Transition10/1
  Switch Startup ramp Angle then Estimated Angle or QEI/1 -> OL/CL/1

== system PIC32MK_MCPWM_MCLV2_PIM_SingleShunt_R2015b_InternalOpAmp/Switch from OpenLoop to Closed Loop ==
  Speed : Inport
  Abs : Abs
  Delay1 : Delay  DelayLength=1  InitialCondition=[0]
  Logical Operator1 : Logic  Operator=OR  AllPortsSameDT=off  OutDataTypeStr=boolean
  Rate Transition8 : RateTransition  OutPortSampleTime=.01
  Switching Speed (rad/s Electrical) : simulink/Logic and Bit Operations/Compare To Constant  relop=>  const=100  OutDataTypeStr=boolean
  ClosedLoop 0/1 : Outport
  wires:
  Abs/1 -> Switching Speed (rad/s Electrical)/1
  Speed/1 -> Rate Transition8/1
  Rate Transition8/1 -> Abs/1
  Delay1/1 -> Logical Operator1/1, ClosedLoop 0/1/1
  Switching Speed (rad/s Electrical)/1 -> Logical Operator1/2
  Logical Operator1/1 -> Delay1/1

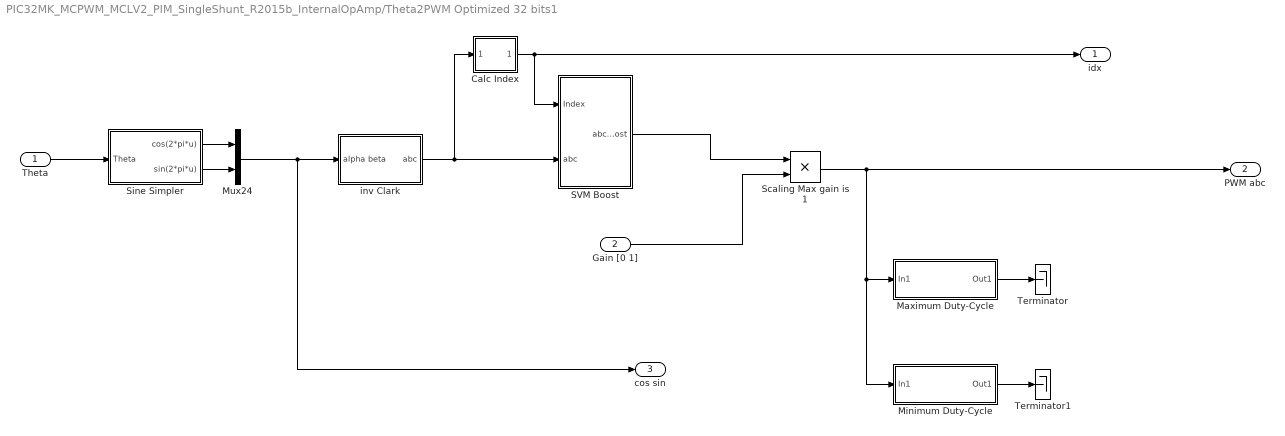
== system PIC32MK_MCPWM_MCLV2_PIM_SingleShunt_R2015b_InternalOpAmp/Theta2PWM Optimized 32 bits1 ==
  Theta : Inport
  Gain [0 1] : Inport  Port=2  OutMax=[PWM1max/2]
  Calc Index : Subsystem
  Maximum Duty-Cycle : Subsystem
  Minimum Duty-Cycle : Subsystem
  Mux24 : Mux  Inputs=2
  SVM Boost : Subsystem
  Scaling Max gain is 1 : Product  Inputs=**  OutDataTypeStr=double
  Sine Simpler : Subsystem
  Terminator : Terminator
  Terminator1 : Terminator
  inv Clark : Subsystem
  idx : Outport
  PWM abc : Outport  Port=2
  cos sin : Outport  Port=3
  wires:
  Mux24/1 -> inv Clark/1(alpha beta), cos sin/1
  SVM Boost/1(abc boost) -> Scaling Max gain is 1/1
  Sine Simpler/2(sin(2*pi*u)) -> Mux24/2
  Sine Simpler/1(cos(2*pi*u)) -> Mux24/1
  Theta/1 -> Sine Simpler/1(Theta)
  inv Clark/1(abc) -> SVM Boost/2(abc), Calc Index/1(In1)
  Calc Index/1(Idx) -> idx/1, SVM Boost/1(Index)
  Gain [0 1]/1 -> Scaling Max gain is 1/2
  Maximum Duty-Cycle/1(Out1) -> Terminator/1
  Minimum Duty-Cycle/1(Out1) -> Terminator1/1
  Scaling Max gain is 1/1 -> PWM abc/1, Maximum Duty-Cycle/1(In1), Minimum Duty-Cycle/1(In1)

== system PIC32MK_MCPWM_MCLV2_PIM_SingleShunt_R2015b_InternalOpAmp/PWM SingleShunt/Build Complementary ==
  Original : Inport
  Modified : Inport  Port=2
  Demux2 : Demux  Outputs=3
  Demux7 : Demux  Outputs=3
  Mux2 : Mux  Inputs=6
  Scope6 : Scope  NumInputPorts=2
  Sum7 : Sum  Inputs=-+
  Sum8 : Sum
  Modified Complementary : Outport
  wires:
  Demux7/3 -> Mux2/6
  Demux7/2 -> Mux2/4
  Demux2/3 -> Mux2/5
  Demux2/2 -> Mux2/3
  Demux7/1 -> Mux2/2
  Demux2/1 -> Mux2/1
  Original/1 -> Sum8/2, Sum7/2
  Modified/1 -> Sum7/1, Demux2/1, Scope6/1
  Mux2/1 -> Modified Complementary/1
  Sum8/1 -> Demux7/1, Scope6/2
  Sum7/1 -> Sum8/1

== system PIC32MK_MCPWM_MCLV2_PIM_SingleShunt_R2015b_InternalOpAmp/PWM SingleShunt/Clamp Not fully ok ==
  In1 : Inport
  Demux2 : Demux  Outputs=3
  Mux1 : Mux  Inputs=3
  Saturation1 : Saturate  UpperLimit=1  LowerLimit=-inf
  Saturation2 : Saturate  UpperLimit=inf  LowerLimit=-1
  Sum : Sum  Inputs=+-
  Sum1 : Sum  Inputs=+-
  Sum2 : Sum  Inputs=-+-
  Out1 : Outport
  wires:
  Demux2/2 -> Sum2/2
  Sum2/1 -> Mux1/2
  Sum1/1 -> Sum2/3
  Sum/1 -> Sum2/1
  Saturation1/1 -> Mux1/1, Sum/2
  Demux2/3 -> Saturation2/1, Sum1/1
  Saturation2/1 -> Mux1/3, Sum1/2
  Demux2/1 -> Saturation1/1, Sum/1
  In1/1 -> Demux2/1
  Mux1/1 -> Out1/1

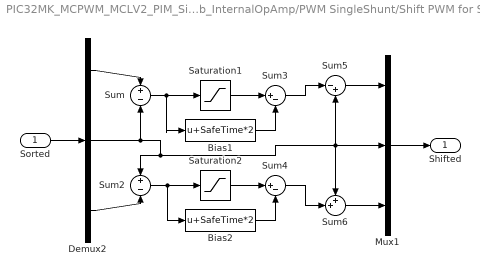
== system PIC32MK_MCPWM_MCLV2_PIM_SingleShunt_R2015b_InternalOpAmp/PWM SingleShunt/Shift PWM for Single Shunt Trig ==
  Sorted : Inport
  Bias1 : Bias  Bias=SafeTime*2
  Bias2 : Bias  Bias=SafeTime*2
  Demux2 : Demux  Outputs=3
  Mux1 : Mux  Inputs=3
  Saturation1 : Saturate  UpperLimit=SafeTime*2  LowerLimit=-inf
  Saturation2 : Saturate  UpperLimit=SafeTime*2  LowerLimit=-inf
  Sum : Sum  Inputs=+-
  Sum2 : Sum  Inputs=+-
  Sum3 : Sum  Inputs=|+-
  Sum4 : Sum  Inputs=|+-
  Sum5 : Sum  Inputs=|-+
  Sum6 : Sum  Inputs=++|
  Shifted : Outport
  wires:
  Sorted/1 -> Demux2/1
  Mux1/1 -> Shifted/1
  Sum4/1 -> Sum6/2
  Bias2/1 -> Sum4/2
  Bias1/1 -> Sum3/2
  Sum5/1 -> Mux1/1
  Sum6/1 -> Mux1/3
  Sum3/1 -> Sum5/1
  Saturation2/1 -> Sum4/1
  Saturation1/1 -> Sum3/1
  Sum2/1 -> Saturation2/1, Bias2/1
  Sum/1 -> Saturation1/1, Bias1/1
  Demux2/3 -> Sum2/2
  Demux2/2 -> Sum/2, Sum5/2, Sum6/1, Mux1/2, Sum2/1
  Demux2/1 -> Sum/1

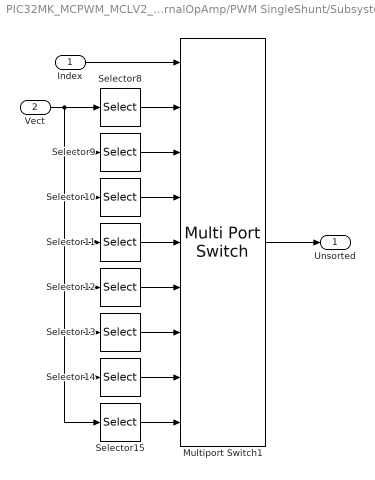
== system PIC32MK_MCPWM_MCLV2_PIM_SingleShunt_R2015b_InternalOpAmp/PWM SingleShunt/Subsystem ==
  Index : Inport
  Vect : Inport  Port=2
  Multiport Switch1 : MultiPortSwitch  DataPortOrder=Zero-based contiguous  Inputs=8  DiagnosticForDefault=None
  Selector10 : Selector  InputPortWidth=3  IndexOptions=Index vector (dialog)  Indices=[1 2 3]  OutputSizes=1
  Selector11 : Selector  InputPortWidth=3  IndexOptions=Index vector (dialog)  Indices=[2 1 3]  OutputSizes=1
  Selector12 : Selector  InputPortWidth=3  IndexOptions=Index vector (dialog)  Indices=[2 3 1]  OutputSizes=1
  Selector13 : Selector  InputPortWidth=3  IndexOptions=Index vector (dialog)  Indices=[1 2 3]  OutputSizes=1
  Selector14 : Selector  InputPortWidth=3  IndexOptions=Index vector (dialog)  Indices=[1 3 2]  OutputSizes=1
  Selector15 : Selector  InputPortWidth=3  IndexOptions=Index vector (dialog)  Indices=[1 2 3]  OutputSizes=1
  Selector8 : Selector  InputPortWidth=3  IndexOptions=Index vector (dialog)  Indices=[3 2 1]  OutputSizes=1
  Selector9 : Selector  InputPortWidth=3  IndexOptions=Index vector (dialog)  Indices=[3 1 2]  OutputSizes=1
  Unsorted : Outport
  wires:
  Index/1 -> Multiport Switch1/1
  Vect/1 -> Selector8/1, Selector15/1, Selector14/1, Selector13/1, Selector12/1, Selector11/1, Selector10/1, Selector9/1
  Multiport Switch1/1 -> Unsorted/1
  Selector8/1 -> Multiport Switch1/2
  Selector11/1 -> Multiport Switch1/5
  Selector12/1 -> Multiport Switch1/6
  Selector14/1 -> Multiport Switch1/8
  Selector13/1 -> Multiport Switch1/7
  Selector10/1 -> Multiport Switch1/4
  Selector9/1 -> Multiport Switch1/3
  Selector15/1 -> Multiport Switch1/9

== system PIC32MK_MCPWM_MCLV2_PIM_SingleShunt_R2015b_InternalOpAmp/PWM SingleShunt/Subsystem1 ==
  Index : Inport
  Vect : Inport  Port=2
  Multiport Switch1 : MultiPortSwitch  DataPortOrder=Zero-based contiguous  Inputs=8  DiagnosticForDefault=None
  Selector10 : Selector  InputPortWidth=3  IndexOptions=Index vector (dialog)  Indices=[1 2 3]  OutputSizes=1
  Selector11 : Selector  InputPortWidth=3  IndexOptions=Index vector (dialog)  Indices=[3 1 2]  OutputSizes=1
  Selector12 : Selector  InputPortWidth=3  IndexOptions=Index vector (dialog)  Indices=[2 1 3]  OutputSizes=1
  Selector13 : Selector  InputPortWidth=3  IndexOptions=Index vector (dialog)  Indices=[1 2 3]  OutputSizes=1
  Selector14 : Selector  InputPortWidth=3  IndexOptions=Index vector (dialog)  Indices=[2 3 1]  OutputSizes=1
  Selector15 : Selector  InputPortWidth=3  IndexOptions=Index vector (dialog)  Indices=[3 2 1]  OutputSizes=1
  Selector8 : Selector  InputPortWidth=3  IndexOptions=Index vector (dialog)  Indices=[1 2 3]  OutputSizes=1
  Selector9 : Selector  InputPortWidth=3  IndexOptions=Index vector (dialog)  Indices=[1 3 2]  OutputSizes=1
  Sorted : Outport
  wires:
  Multiport Switch1/1 -> Sorted/1
  Index/1 -> Multiport Switch1/1
  Selector12/1 -> Multiport Switch1/5
  Selector8/1 -> Multiport Switch1/9
  Selector14/1 -> Multiport Switch1/3
  Selector15/1 -> Multiport Switch1/2
  Selector10/1 -> Multiport Switch1/7
  Selector11/1 -> Multiport Switch1/6
  Selector9/1 -> Multiport Switch1/8
  Selector13/1 -> Multiport Switch1/4
  Vect/1 -> Selector15/1, Selector8/1, Selector9/1, Selector10/1, Selector11/1, Selector12/1, Selector13/1, Selector14/1

== system PIC32MK_MCPWM_MCLV2_PIM_SingleShunt_R2015b_InternalOpAmp/Sensors1/Reconstruct Ia Ib ==
  Index : Inport
  I : Inport  Port=2
  Demux1 : Demux  Outputs=2
  Gain1 : Gain  Gain=-1  OutDataTypeStr=Inherit: Same as input
  Multiport Switch1 : MultiPortSwitch  DataPortOrder=Zero-based contiguous  Inputs=8  DiagnosticForDefault=None
  Multiport Switch2 : MultiPortSwitch  DataPortOrder=Zero-based contiguous  Inputs=8  DiagnosticForDefault=None
  Mux : Mux  Inputs=2
  Sum1 : Sum  Inputs=+-
  Ia Ib : Outport
  wires:
  I/1 -> Demux1/1
  Index/1 -> Multiport Switch1/1, Multiport Switch2/1
  Demux1/2 -> Sum1/2, Multiport Switch2/6, Multiport Switch2/8, Multiport Switch1/3, Multiport Switch1/2
  Demux1/1 -> Sum1/1, Gain1/1
  Mux/1 -> Ia Ib/1
  Multiport Switch2/1 -> Mux/2
  Multiport Switch1/1 -> Mux/1
  Gain1/1 -> Multiport Switch2/5, Multiport Switch2/3, Multiport Switch1/9, Multiport Switch1/8
  Sum1/1 -> Multiport Switch1/5, Multiport Switch1/6, Multiport Switch2/2, Multiport Switch2/9

== system PIC32MK_MCPWM_MCLV2_PIM_SingleShunt_R2015b_InternalOpAmp/Sensors1/Reconstruct Ia Ib1 ==
  Index : Inport
  I : Inport  Port=2
  Demux1 : Demux  Outputs=2
  Gain1 : Gain  Gain=-1  OutDataTypeStr=Inherit: Same as input
  Multiport Switch1 : MultiPortSwitch  DataPortOrder=Zero-based contiguous  Inputs=8  DiagnosticForDefault=None
  Multiport Switch2 : MultiPortSwitch  DataPortOrder=Zero-based contiguous  Inputs=8  DiagnosticForDefault=None
  Mux : Mux  Inputs=2
  Sum1 : Sum  Inputs=+-
  Ia Ib : Outport
  wires:
  Sum1/1 -> Multiport Switch2/9, Multiport Switch2/2, Multiport Switch1/6, Multiport Switch1/5
  Gain1/1 -> Multiport Switch1/8, Multiport Switch1/9, Multiport Switch2/3, Multiport Switch2/5
  Multiport Switch1/1 -> Mux/1
  Multiport Switch2/1 -> Mux/2
  Mux/1 -> Ia Ib/1
  Demux1/1 -> Gain1/1, Sum1/1
  Demux1/2 -> Multiport Switch1/2, Multiport Switch1/3, Multiport Switch2/8, Multiport Switch2/6, Sum1/2
  Index/1 -> Multiport Switch2/1, Multiport Switch1/1
  I/1 -> Demux1/1

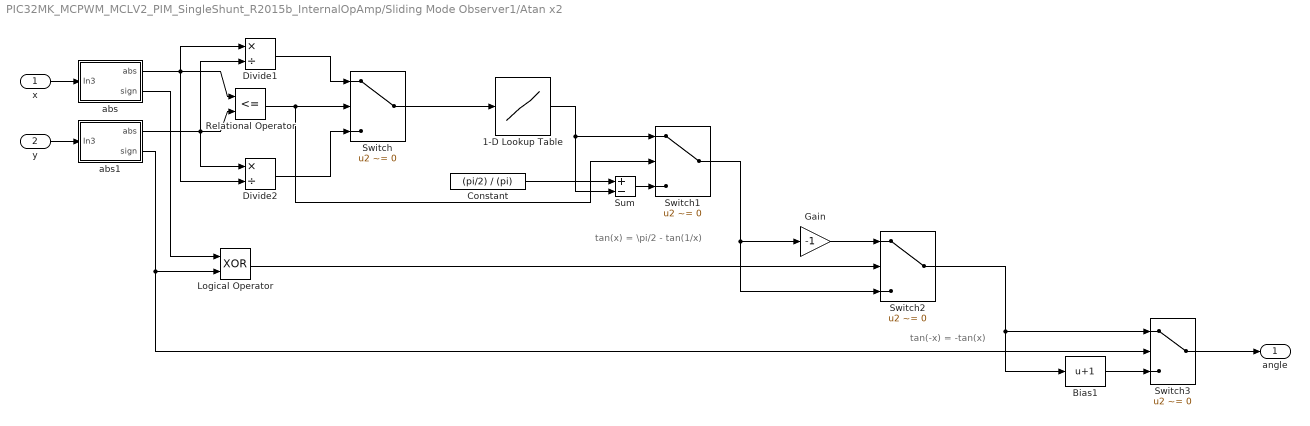
== system PIC32MK_MCPWM_MCLV2_PIM_SingleShunt_R2015b_InternalOpAmp/Sliding Mode Observer1/Atan x2 ==
  note: tan(x) = \pi/2 - tan(1/x)
  note: tan(-x) = -tan(x)
  x : Inport
  y : Inport  Port=2
  1-D Lookup Table : Lookup_n-D  NumberOfTableDimensions=1  BreakpointsSpecification=Even spacing  BreakpointsForDimension1=[0:2^-8:1]  BreakpointsForDimension1FirstPoint=0  BreakpointsForDimension1Spacing=2^-8  IndexSearchMethod=Evenly spaced points  BeginIndexSearchUsingPreviousIndexResult=on  Table=atan([0:2^-8:1])/(pi)  TableDataTypeStr=fixdt(1,32,31)  InterpMethod=Flat  ExtrapMethod=Clip  RemoveProtectionInput=on  UseLastTableValue=on  OutDataTypeStr=fixdt(1,32,31)  RndMeth=Simplest  InputSameDT=on  LockScale=on
  Bias1 : Bias  Bias=1
  Constant : Constant  Value=(pi/2) / (pi)  OutDataTypeStr=Inherit: Inherit via back propagation
  Divide1 : Product  Inputs=*/  OutDataTypeStr=fixdt(0,16,15)
  Divide2 : Product  Inputs=*/  OutDataTypeStr=fixdt(0,16,15)
  Gain : Gain  Gain=-1  OutDataTypeStr=Inherit: Same as input
  Logical Operator : Logic  Operator=XOR  AllPortsSameDT=off  OutDataTypeStr=boolean
  Relational Operator : RelationalOperator  Operator=<=  OutDataTypeStr=boolean
  Sum : Sum  Inputs=+-
  Switch{,1..3} (4 alike) : Switch  Criteria=u2 ~= 0
  abs : Subsystem
  abs1 : Subsystem
  angle : Outport
  wires:
  Gain/1 -> Switch2/1
  Bias1/1 -> Switch3/3
  Switch3/1 -> angle/1
  Switch2/1 -> Switch3/1, Bias1/1
  Relational Operator/1 -> Switch/2, Switch1/2
  Divide2/1 -> Switch/3
  Divide1/1 -> Switch/1
  Switch/1 -> 1-D Lookup Table/1
  1-D Lookup Table/1 -> Switch1/1, Sum/2
  Constant/1 -> Sum/1
  Sum/1 -> Switch1/3
  abs/1(abs) -> Relational Operator/1, Divide1/1, Divide2/2
  x/1 -> abs/1(In3)
  abs1/1(abs) -> Relational Operator/2, Divide2/1, Divide1/2
  y/1 -> abs1/1(In3)
  abs/2(sign) -> Logical Operator/1
  abs1/2(sign) -> Logical Operator/2, Switch3/2
  Logical Operator/1 -> Switch2/2
  Switch1/1 -> Gain/1, Switch2/3

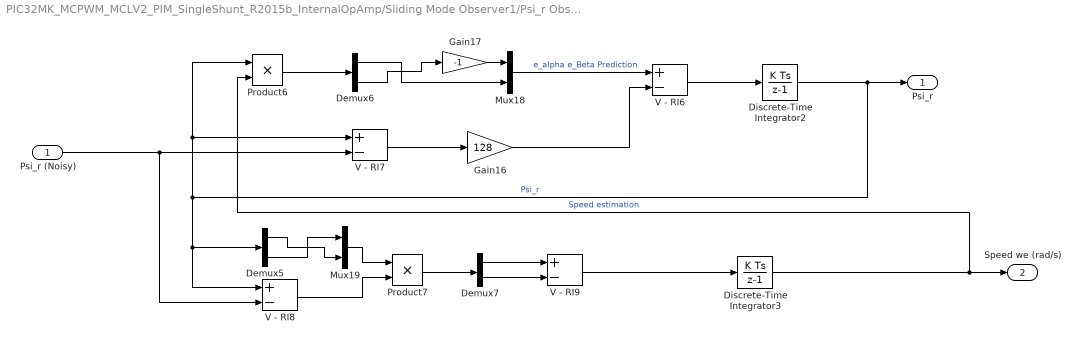
== system PIC32MK_MCPWM_MCLV2_PIM_SingleShunt_R2015b_InternalOpAmp/Sliding Mode Observer1/Psi_r Observer Speed Observer2 ==
  Psi_r (Noisy) : Inport
  Demux5 : Demux  Outputs=2
  Demux6 : Demux  Outputs=2
  Demux7 : Demux  Outputs=2
  Discrete-Time Integrator2 : DiscreteIntegrator  gainval=1  SampleTime=-1  OutMin=-24  OutMax=24  RndMeth=Zero  UpperSaturationLimit=15  LowerSaturationLimit=-15  ICPrevOutput=DiscIntNeverNeededParam  ICPrevScaledInput=DiscIntNeverNeededParam
  Discrete-Time Integrator3 : DiscreteIntegrator  gainval=1000  SampleTime=-1  OutMin=-5300 * 5 * (2*pi) / 60  OutMax=5300 * 5 * (2*pi) / 60  RndMeth=Zero  StateIdentifier=Speed  ICPrevOutput=DiscIntNeverNeededParam  ICPrevScaledInput=DiscIntNeverNeededParam
  Gain16 : Gain  Gain=128  OutMin=[-24*2*128]  OutMax=[24*2*128]  RndMeth=Zero
  Gain17 : Gain  Gain=-1  OutDataTypeStr=Inherit: Same as input
  Mux18 : Mux  Inputs=2
  Mux19 : Mux  Inputs=2
  Product6 : Product  RndMeth=Zero
  Product7 : Product  OutMin=[-24*24]  OutMax=24*24  RndMeth=Zero
  V - RI6 : Sum  Inputs=+-  OutDataTypeStr=Inherit: Same as accumulator  RndMeth=Zero
  V - RI7 : Sum  Inputs=+-  OutMin=[-24*2]  OutMax=[24*2]  RndMeth=Zero
  V - RI8 : Sum  Inputs=+-  OutDataTypeStr=Inherit: Same as accumulator  RndMeth=Zero
  V - RI9 : Sum  Inputs=+-  OutMin=[-24*24*2]  OutMax=[-24*24*2]  RndMeth=Zero  InputSameDT=on
  Psi_r : Outport
  Speed we (rad/s) : Outport  Port=2
  wires:
  V - RI9/1 -> Discrete-Time Integrator3/1
  V - RI6/1 -> Discrete-Time Integrator2/1
  V - RI7/1 -> Gain16/1
  Mux18/1 -> V - RI6/1  "e_alpha e_Beta Prediction"
  Demux5/2 -> Mux19/1
  Mux19/1 -> Product7/1
  V - RI8/1 -> Product7/2
  Product7/1 -> Demux7/1
  Demux7/1 -> V - RI9/1
  Demux7/2 -> V - RI9/2
  Product6/1 -> Demux6/1
  Gain17/1 -> Mux18/1
  Discrete-Time Integrator3/1 -> Product6/2, Speed we (rad/s)/1  "Speed estimation"
  Demux6/1 -> Mux18/2
  Psi_r (Noisy)/1 -> V - RI8/2, V - RI7/2
  Demux6/2 -> Gain17/1
  Demux5/1 -> Mux19/2
  Discrete-Time Integrator2/1 -> Psi_r/1, Product6/1, V - RI7/1, V - RI8/1, Demux5/1  "Psi_r"
  Gain16/1 -> V - RI6/2

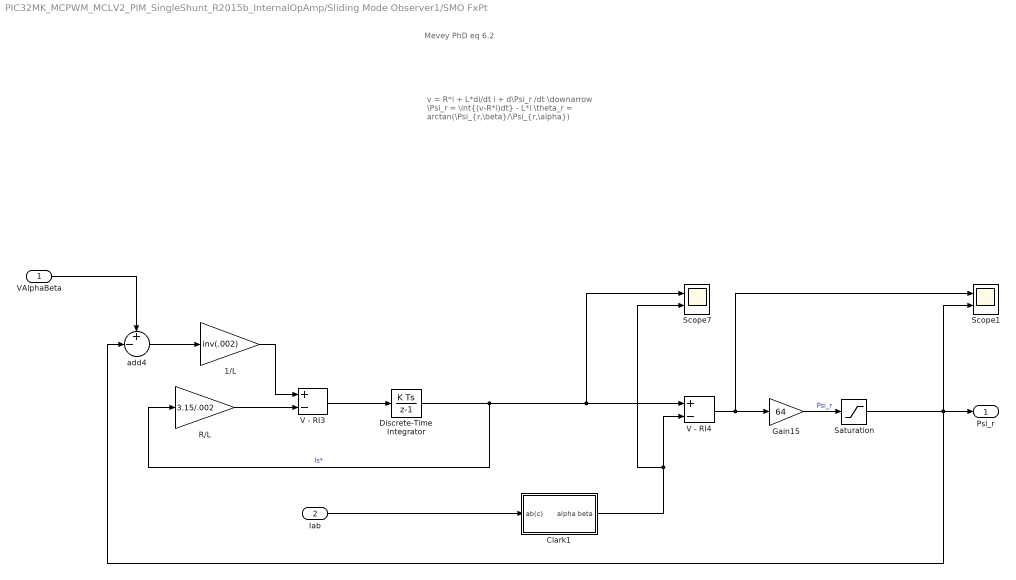
== system PIC32MK_MCPWM_MCLV2_PIM_SingleShunt_R2015b_InternalOpAmp/Sliding Mode Observer1/SMO FxPt ==
  note: v = R*i + L*di/dt i + d\Psi_r /dt
      | \downarrow
      | \Psi_r = \int{(v-R*i)dt} - L*i
      | \theta_r = arctan(\Psi_{r,\beta}/\Psi_{r,\alpha})
  note: Mevey PhD eq 6.2
  VAlphaBeta : Inport
  Iab : Inport  Port=2
  1/L : Gain  Gain=inv(.002)  OutMin=[-24] * inv(.002) *2  OutMax=[24] * inv(.002) *2  RndMeth=Zero
  Clark1 : Subsystem
  Discrete-Time Integrator : DiscreteIntegrator  SampleTime=-1  OutMin=[-4.4]  OutMax=[4.4]  RndMeth=Zero  ICPrevOutput=DiscIntNeverNeededParam  ICPrevScaledInput=DiscIntNeverNeededParam
  Gain15 : Gain  Gain=64  OutMin=[-24]  OutMax=[24]  RndMeth=Zero
  R/L : Gain  Gain=3.15/.002  OutMin=-4.4*3.15/0.002  OutMax=4.4*3.15/0.002  RndMeth=Zero
  Saturation : Saturate  UpperLimit=32  LowerLimit=-32
  Scope1 : Scope  NumInputPorts=2
  Scope7 : Scope  NumInputPorts=2
  V - RI3 : Sum  Inputs=+-  OutDataTypeStr=Inherit: Same as accumulator  RndMeth=Zero
  V - RI4 : Sum  Inputs=+-  OutMin=-4.4  OutMax=4.4  RndMeth=Zero
  add4 : Sum  Inputs=+-|  OutDataTypeStr=Inherit: Same as accumulator  RndMeth=Zero
  Psi_r : Outport
  wires:
  Saturation/1 -> Psi_r/1, add4/2, Scope1/2
  Gain15/1 -> Saturation/1  "Psi_r"
  Clark1/1(alpha beta) -> Scope7/2, V - RI4/2
  Iab/1 -> Clark1/1(ab(c))
  V - RI4/1 -> Gain15/1, Scope1/1
  Discrete-Time Integrator/1 -> Scope7/1, V - RI4/1, R/L/1  "Is*"
  V - RI3/1 -> Discrete-Time Integrator/1
  VAlphaBeta/1 -> add4/1
  add4/1 -> 1/L/1
  R/L/1 -> V - RI3/2
  1/L/1 -> V - RI3/1

== system PIC32MK_MCPWM_MCLV2_PIM_SingleShunt_R2015b_InternalOpAmp/Theta2PWM Optimized 32 bits1/Calc Index ==
  In1 : Inport
  Bitwise Operator1 : simulink/Logic and Bit Operations/Bitwise Operator  logicop=OR  UseBitMask=off  NumInputPorts=3  BitMask=bin2dec('11011001')  BitMaskRealWorld=Stored Integer
  Data Type Conversion : DataTypeConversion  OutDataTypeStr=uint32  ConvertRealWorld=Stored Integer (SI)
  Demux1 : Demux  Outputs=3
  Gain6 : Gain  Gain=4  OutDataTypeStr=Inherit: Same as input
  Gain7 : Gain  Gain=2  OutDataTypeStr=Inherit: Same as input
  Relational Operator1 : RelationalOperator  Operator=>  OutDataTypeStr=fixdt(0,32)
  Relational Operator2 : RelationalOperator  Operator=>  OutDataTypeStr=fixdt(0,32)
  Relational Operator3 : RelationalOperator  Operator=>  OutDataTypeStr=fixdt(0,32)
  Idx : Outport
  wires:
  Data Type Conversion/1 -> Idx/1
  In1/1 -> Demux1/1
  Bitwise Operator1/1 -> Data Type Conversion/1
  Demux1/1 -> Relational Operator3/1, Relational Operator1/1
  Relational Operator1/1 -> Gain7/1
  Demux1/3 -> Relational Operator1/2, Relational Operator2/2
  Demux1/2 -> Relational Operator3/2, Relational Operator2/1
  Relational Operator3/1 -> Gain6/1
  Relational Operator2/1 -> Bitwise Operator1/3
  Gain6/1 -> Bitwise Operator1/1
  Gain7/1 -> Bitwise Operator1/2

== system PIC32MK_MCPWM_MCLV2_PIM_SingleShunt_R2015b_InternalOpAmp/Theta2PWM Optimized 32 bits1/Maximum Duty-Cycle ==
  In1 : Inport
  Constant1 : Constant  Value=PWM1max  OutDataTypeStr=uint16
  MinMax1 : MinMax  Function=max  OutDataTypeStr=int16  InputSameDT=on
  Sum1 : Sum  Inputs=+-  AccumDataTypeStr=uint16  OutDataTypeStr=Inherit: Same as accumulator  RndMeth=Simplest
  Sum2 : Sum  Inputs=|++  AccumDataTypeStr=uint16  OutDataTypeStr=Inherit: Same as accumulator  RndMeth=Simplest
  Out1 : Outport
  wires:
  Constant1/1 -> Sum1/1
  MinMax1/1 -> Sum1/2
  In1/1 -> Sum2/1, MinMax1/1
  Sum2/1 -> Out1/1
  Sum1/1 -> Sum2/2

== system PIC32MK_MCPWM_MCLV2_PIM_SingleShunt_R2015b_InternalOpAmp/Theta2PWM Optimized 32 bits1/Minimum Duty-Cycle ==
  In1 : Inport
  Bias : Bias  Bias=-round( (2e-6/5e-5) *PWM1max )
  MinMax1 : MinMax  OutDataTypeStr=int16  InputSameDT=on
  Sum2 : Sum  Inputs=|+-  AccumDataTypeStr=uint16  OutDataTypeStr=Inherit: Same as accumulator  RndMeth=Simplest
  Out1 : Outport
  wires:
  In1/1 -> MinMax1/1, Sum2/1
  Sum2/1 -> Out1/1
  MinMax1/1 -> Bias/1
  Bias/1 -> Sum2/2

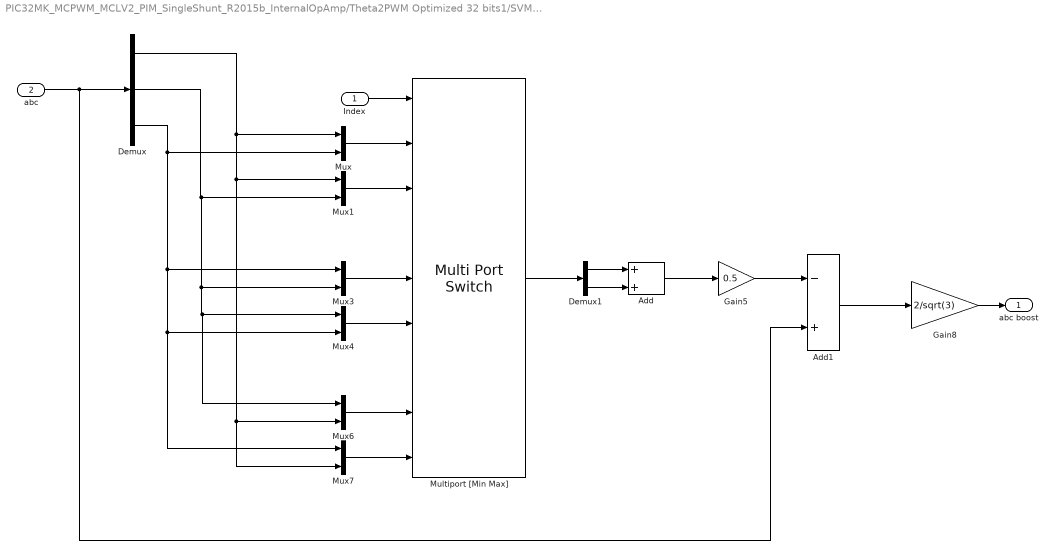
== system PIC32MK_MCPWM_MCLV2_PIM_SingleShunt_R2015b_InternalOpAmp/Theta2PWM Optimized 32 bits1/SVM Boost ==
  Index : Inport
  abc : Inport  Port=2
  Add : Sum  OutDataTypeStr=Inherit: Same as accumulator  RndMeth=Zero
  Add1 : Sum  Inputs=-+  RndMeth=Zero  OutDataTypeStr=Inherit: Same as first input
  Demux : Demux  Outputs=3
  Demux1 : Demux  Outputs=2
  Gain5 : Gain  Gain=0.5  RndMeth=Zero  OutDataTypeStr=Inherit: Same as input
  Gain8 : Gain  Gain=2/sqrt(3)  RndMeth=Zero  ParamDataTypeStr=Inherit: Same as input
  Multiport [Min Max] : MultiPortSwitch  DataPortOrder=Zero-based contiguous  Inputs=8  DiagnosticForDefault=None
  Mux{,1,3..4,6..7} (6 alike) : Mux  Inputs=2
  abc boost : Outport
  wires:
  Add/1 -> Gain5/1
  Gain5/1 -> Add1/1
  Add1/1 -> Gain8/1
  abc/1 -> Add1/2, Demux/1
  Gain8/1 -> abc boost/1
  Index/1 -> Multiport [Min Max]/1
  Mux/1 -> Multiport [Min Max]/2
  Mux1/1 -> Multiport [Min Max]/3
  Mux3/1 -> Multiport [Min Max]/5
  Mux4/1 -> Multiport [Min Max]/6
  Mux6/1 -> Multiport [Min Max]/8
  Mux7/1 -> Multiport [Min Max]/9
  Demux/1 -> Mux7/2, Mux6/2, Mux1/1, Mux/1
  Demux/3 -> Mux/2, Mux3/1, Mux4/2, Mux7/1
  Demux/2 -> Mux6/1, Mux4/1, Mux3/2, Mux1/2
  Multiport [Min Max]/1 -> Demux1/1
  Demux1/1 -> Add/1
  Demux1/2 -> Add/2

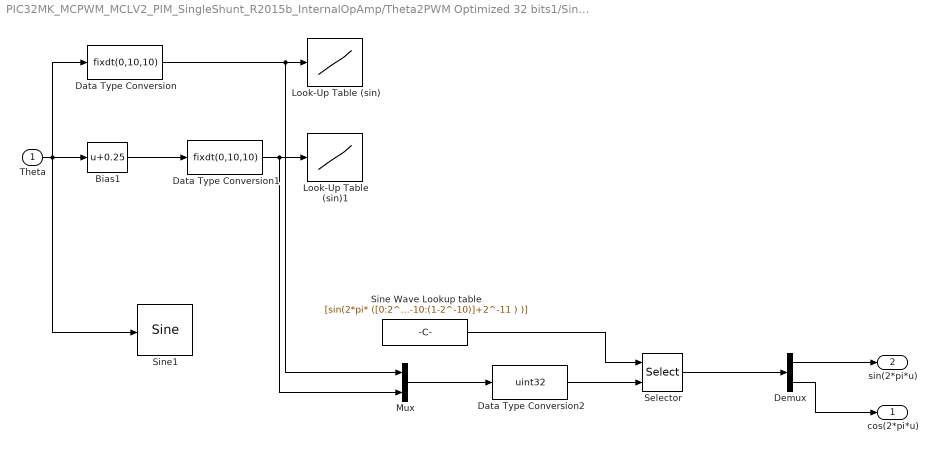
== system PIC32MK_MCPWM_MCLV2_PIM_SingleShunt_R2015b_InternalOpAmp/Theta2PWM Optimized 32 bits1/Sine Simpler ==
  Theta : Inport
  Bias1 : Bias  Bias=0.25
  Data Type Conversion : DataTypeConversion  OutDataTypeStr=fixdt(0,10,10)
  Data Type Conversion1 : DataTypeConversion  OutDataTypeStr=fixdt(0,10,10)
  Data Type Conversion2 : DataTypeConversion  OutDataTypeStr=uint32  ConvertRealWorld=Stored Integer (SI)
  Demux : Demux  Outputs=2
  Look-Up Table (sin) : Lookup_n-D  NumberOfTableDimensions=1  BreakpointsSpecification=Even spacing  BreakpointsForDimension1=XData  BreakpointsForDimension1FirstPoint=0  BreakpointsForDimension1Spacing=2^-10  IndexSearchMethod=Evenly spaced points  Table=sin(2*pi* ([0:2^-10:(1-2^-10)]+2^-11 ) )  InterpMethod=Flat  ExtrapMethod=Clip  RemoveProtectionInput=on  InternalRulePriority=Speed  OutDataTypeStr=fixdt(1, 32, 30)  RndMeth=Zero  LockScale=on
  Look-Up Table (sin)1 : Lookup_n-D  NumberOfTableDimensions=1  BreakpointsSpecification=Even spacing  BreakpointsForDimension1=XData  BreakpointsForDimension1FirstPoint=0  BreakpointsForDimension1Spacing=2^-10  IndexSearchMethod=Evenly spaced points  Table=sin(2*pi* ([0:2^-10:(1-2^-10)]+2^-11 ) )  InterpMethod=Flat  ExtrapMethod=Clip  RemoveProtectionInput=on  InternalRulePriority=Speed  OutDataTypeStr=fixdt(1, 32, 30)  RndMeth=Zero  LockScale=on
  Mux : Mux  Inputs=2
  Selector : Selector  IndexMode=Zero-based  InputPortWidth=1024  IndexOptions=Index vector (port)  Indices=[1 3]  OutputSizes=1
  Sine Wave Lookup table : Constant  Value=[sin(2*pi* ([0:2^-10:(1-2^-10)]+2^-11 ) )]  OutDataTypeStr=double
  Sine1 : simulink/Lookup Tables/Sine  Formula=sin(2*pi*u) and cos(2*pi*u)  NumDataPoints=(2^5)+1  OutputWordLength=16  InternalRulePriority=Speed
  cos(2*pi*u) : Outport
  sin(2*pi*u) : Outport  Port=2
  wires:
  Demux/2 -> cos(2*pi*u)/1
  Demux/1 -> sin(2*pi*u)/1
  Selector/1 -> Demux/1
  Data Type Conversion2/1 -> Selector/2
  Mux/1 -> Data Type Conversion2/1
  Sine Wave Lookup table/1 -> Selector/1
  Data Type Conversion1/1 -> Look-Up Table (sin)1/1, Mux/2
  Data Type Conversion/1 -> Look-Up Table (sin)/1, Mux/1
  Theta/1 -> Sine1/1, Data Type Conversion/1, Bias1/1
  Bias1/1 -> Data Type Conversion1/1

== system PIC32MK_MCPWM_MCLV2_PIM_SingleShunt_R2015b_InternalOpAmp/Theta2PWM Optimized 32 bits1/inv Clark ==
  note: Transposed version is better optimized with DSP (optional)
      | No impact on no DSP version
  note: k = 2/3 : invariant Magnitude
  alpha beta : Inport
  Clarke1 : Product  Multiplication=Matrix(*)  RndMeth=Simplest  OutDataTypeStr=Inherit: Same as first input
  Constant Magnitude : Constant  Value=[1 0 ; -1/2 sqrt(3)/2 ;-1/2 -sqrt(3)/2]'  OutDataTypeStr=Inherit: Inherit via back propagation  SampleTime=-1
  Demux : Demux  Outputs=2
  Gain : Gain  Gain=sqrt(3)/2  OutDataTypeStr=Inherit: Inherit via back propagation  RndMeth=Zero
  Gain3 : Gain  Gain=-1/2  OutDataTypeStr=Inherit: Inherit via back propagation  RndMeth=Zero
  Math Function : Math  Operator=transpose  SaturateOnIntegerOverflow=on
  Math Function1 : Math  Operator=transpose  SaturateOnIntegerOverflow=on
  Mux : Mux  Inputs=3
  Sum : Sum  RndMeth=Zero  OutDataTypeStr=Inherit: Same as first input
  Sum1 : Sum  Inputs=+-  RndMeth=Zero  SaturateOnIntegerOverflow=on  OutDataTypeStr=Inherit: Same as first input
  abc : Outport
  wires:
  Demux/1 -> Gain3/1, Mux/1
  Demux/2 -> Gain/1
  Constant Magnitude/1 -> Clarke1/2
  alpha beta/1 -> Math Function/1, Demux/1
  Gain/1 -> Sum1/2, Sum/1
  Sum/1 -> Mux/2
  Sum1/1 -> Mux/3
  Gain3/1 -> Sum1/1, Sum/2
  Clarke1/1 -> Math Function1/1
  Math Function/1 -> Clarke1/1
  Mux/1 -> abc/1
